simulink model "regulator_obserwator"  (R2022a)
settings: Solver=VariableStepAuto  StartTime=0.0  StopTime=10.0  RelTol=1e-3
values from neighbouring files (symbols this model uses):
  k1 = -3*sb - 33    (= -30)    [dane.m]
  k2 = 3*sb^2 -362    (= -359)    [dane.m]
  k3 = -sb^3 -1320    (= -1319)    [dane.m]
  L1 = -(14149*so)/30 - (781*so^2)/15 - (347*so^3)/180 - 130493/90    (= 415.827777778)    [dane.m]
  L2 = (77*so^3)/360 + (347*so^2)/60 + (781*so)/15 + 14149/90    (= -44.4138888889)    [dane.m]
  L3 = -(347*so)/60 - (77*so^2)/120 - (17*so^3)/720 - 781/45    (= 4.70694444444)    [dane.m]
settings Model: Creator=danie  LastModifiedBy=danie

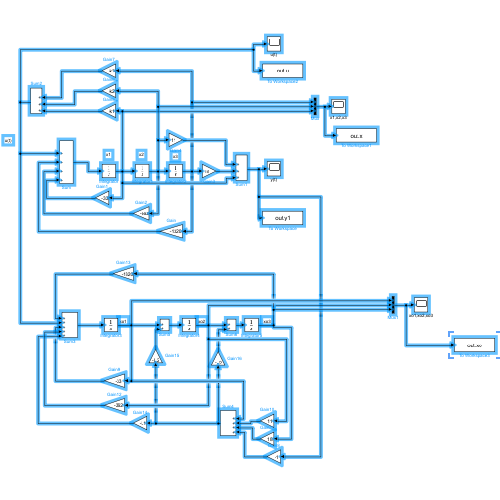
[thumbnail: Simulink's stored preview of the top-level diagram]
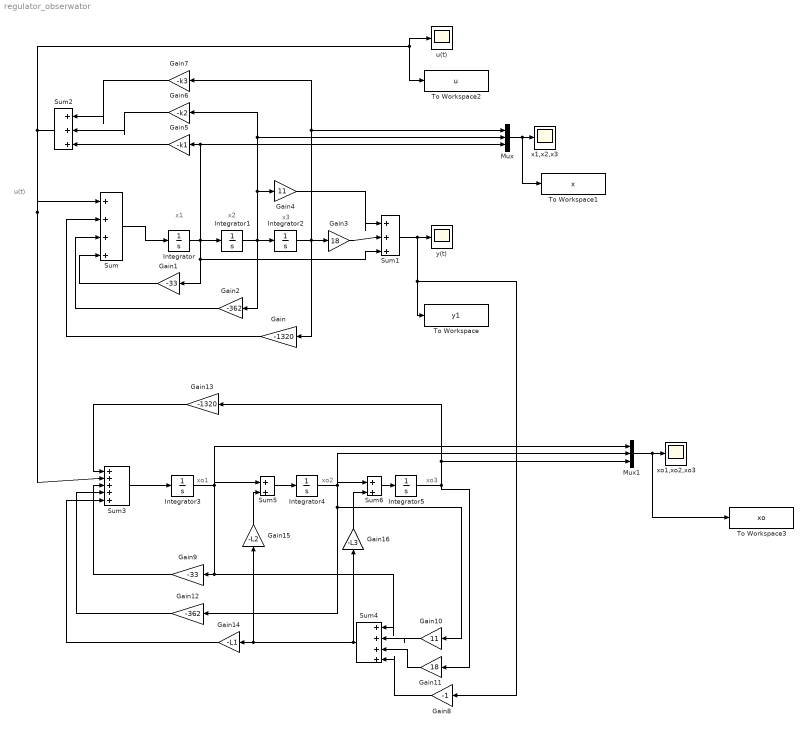
== system regulator_obserwator ==
  note: u(t)
  note: x1
  note: x3
  note: x2
  note: xo2
  note: xo1
  note: xo3
  Gain : Gain  Gain=-1320
  Gain1 : Gain  Gain=-33
  Gain10 : Gain  Gain=11
  Gain11 : Gain  Gain=18
  Gain12 : Gain  Gain=-362
  Gain13 : Gain  Gain=-1320
  Gain14 : Gain  Gain=-L1
  Gain15 : Gain  Gain=-L2
  Gain16 : Gain  Gain=-L3
  Gain2 : Gain  Gain=-362
  Gain3 : Gain  Gain=18
  Gain4 : Gain  Gain=11
  Gain5 : Gain  Gain=-k1
  Gain6 : Gain  Gain=-k2
  Gain7 : Gain  Gain=-k3
  Gain8 : Gain  Gain=-1
  Gain9 : Gain  Gain=-33
  Integrator : Integrator  InitialCondition=3
  Integrator1 : Integrator  InitialCondition=2
  Integrator2 : Integrator  InitialCondition=-3
  Integrator3 : Integrator
  Integrator4 : Integrator
  Integrator5 : Integrator
  Mux : Mux  Inputs=3
  Mux1 : Mux  Inputs=3
  Sum : Sum  Inputs=|++++
  Sum1 : Sum  Inputs=|+++
  Sum2 : Sum  Inputs=|+++
  Sum3 : Sum  Inputs=|+++++
  Sum4 : Sum  Inputs=|++++
  Sum5 : Sum  Inputs=|++
  Sum6 : Sum  Inputs=|++
  To Workspace : ToWorkspace  VariableName=y1  SaveFormat=Structure With Time  SampleTime=-1
  To Workspace1 : ToWorkspace  VariableName=x  SaveFormat=Structure With Time  SampleTime=-1
  To Workspace2 : ToWorkspace  VariableName=u  SaveFormat=Structure With Time  SampleTime=-1
  To Workspace3 : ToWorkspace  VariableName=xo  SaveFormat=Structure With Time  SampleTime=-1
  u(t) : Scope
  x1,x2,x3 : Scope
  xo1,xo2,xo3 : Scope
  y(t) : Scope
  wires:
  Mux/1 -> To Workspace1/1, x1,x2,x3/1
  Gain7/1 -> Sum2/1
  Integrator2/1 -> Gain7/1, Mux/1, Gain/1, Gain3/1
  Gain1/1 -> Sum/4
  Gain3/1 -> Sum1/2
  Gain5/1 -> Sum2/3
  Sum/1 -> Integrator/1
  Gain6/1 -> Sum2/2
  Integrator/1 -> Sum1/3, Gain1/1, Integrator1/1, Mux/3, Gain5/1
  Gain4/1 -> Sum1/1
  Integrator1/1 -> Gain4/1, Gain6/1, Mux/2, Gain2/1, Integrator2/1
  Sum2/1 -> Sum3/2, Sum/1, u(t)/1, To Workspace2/1
  Sum5/1 -> Integrator4/1
  Sum4/1 -> Gain15/1, Gain14/1, Gain16/1
  Gain8/1 -> Sum4/4
  Gain13/1 -> Sum3/1
  Gain11/1 -> Sum4/3
  Gain14/1 -> Sum3/5
  Sum6/1 -> Integrator5/1
  Integrator3/1 -> Sum5/1, Mux1/1, Sum4/1, Gain9/1
  Gain9/1 -> Sum3/3
  Gain10/1 -> Sum4/2
  Gain12/1 -> Sum3/4
  Gain15/1 -> Sum5/2
  Gain16/1 -> Sum6/2
  Integrator4/1 -> Mux1/2, Gain10/1, Gain12/1, Sum6/1
  Sum3/1 -> Integrator3/1
  Integrator5/1 -> Mux1/3, Gain13/1, Gain11/1
  Gain2/1 -> Sum/3
  Gain/1 -> Sum/2
  Sum1/1 -> Gain8/1, To Workspace/1, y(t)/1
  Mux1/1 -> To Workspace3/1, xo1,xo2,xo3/1
